simulink model "cic32"  (R2019a)
settings: Solver=VariableStepAuto  StartTime=0.0  StopTime=10.0  RelTol=1e-3
settings Model: Creator=Wunyje  LastModifiedBy=Wunyje

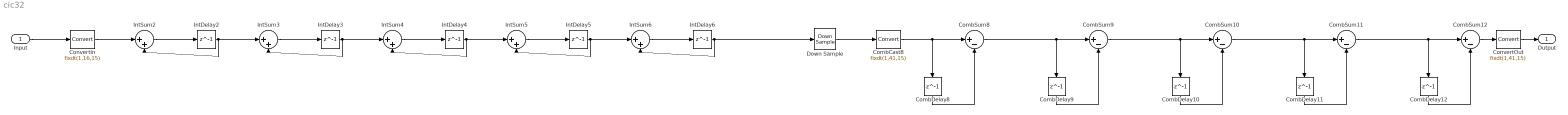
== system cic32 ==
  Input : Inport
  CombCast8 : DataTypeConversion  OutDataTypeStr=fixdt(1,41,15)
  CombDelay{8..12} (5 alike) : Delay  DelayLength=1  InitialCondition=0
  CombSum{8..12} (5 alike) : Sum  Inputs=|+-  AccumDataTypeStr=fixdt(1,41,15)  OutDataTypeStr=fixdt(1,41,15)
  ConvertIn : DataTypeConversion  OutDataTypeStr=fixdt(1,16,15)  RndMeth=Nearest  SaturateOnIntegerOverflow=on
  ConvertOut : DataTypeConversion  OutDataTypeStr=fixdt(1,41,15)
  Down Sample : DownSample  N=32  RateOptions=Allow multirate processing
  IntDelay{2..6} (5 alike) : Delay  DelayLength=1  InitialCondition=0
  IntSum{2..6} (5 alike) : Sum  Inputs=|++  AccumDataTypeStr=fixdt(1,41,15)  OutDataTypeStr=fixdt(1,41,15)
  Output : Outport  VectorParamsAs1DForOutWhenUnconnected=on
  wires:
  IntSum6/1 -> IntDelay6/1
  ConvertOut/1 -> Output/1
  CombDelay12/1 -> CombSum12/2
  Down Sample/1 -> CombCast8/1
  IntDelay2/1 -> IntSum2/2, IntSum3/1
  CombSum9/1 -> CombSum10/1, CombDelay10/1
  CombCast8/1 -> CombSum8/1, CombDelay8/1
  CombDelay10/1 -> CombSum10/2
  CombDelay11/1 -> CombSum11/2
  CombDelay9/1 -> CombSum9/2
  CombSum8/1 -> CombSum9/1, CombDelay9/1
  IntDelay6/1 -> IntSum6/2, Down Sample/1
  CombSum10/1 -> CombSum11/1, CombDelay11/1
  CombSum11/1 -> CombSum12/1, CombDelay12/1
  CombDelay8/1 -> CombSum8/2
  ConvertIn/1 -> IntSum2/1
  CombSum12/1 -> ConvertOut/1
  IntDelay3/1 -> IntSum3/2, IntSum4/1
  IntSum3/1 -> IntDelay3/1
  IntSum5/1 -> IntDelay5/1
  IntDelay5/1 -> IntSum5/2, IntSum6/1
  IntDelay4/1 -> IntSum4/2, IntSum5/1
  IntSum2/1 -> IntDelay2/1
  IntSum4/1 -> IntDelay4/1
  Input/1 -> ConvertIn/1
